simulink library "Cassie_CommandBlock_Library_1"  (R2017b)
settings: Solver=VariableStepAuto  StartTime=0.0  StopTime=10.0  RelTol=1e-3
undefined symbols (not defined in the file): isSim, UserParams
settings Model: Creator=81068  LastModifiedBy=81068

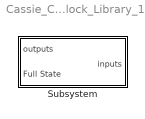
== system Cassie_CommandBlock_Library_1 ==
  Subsystem : Subsystem

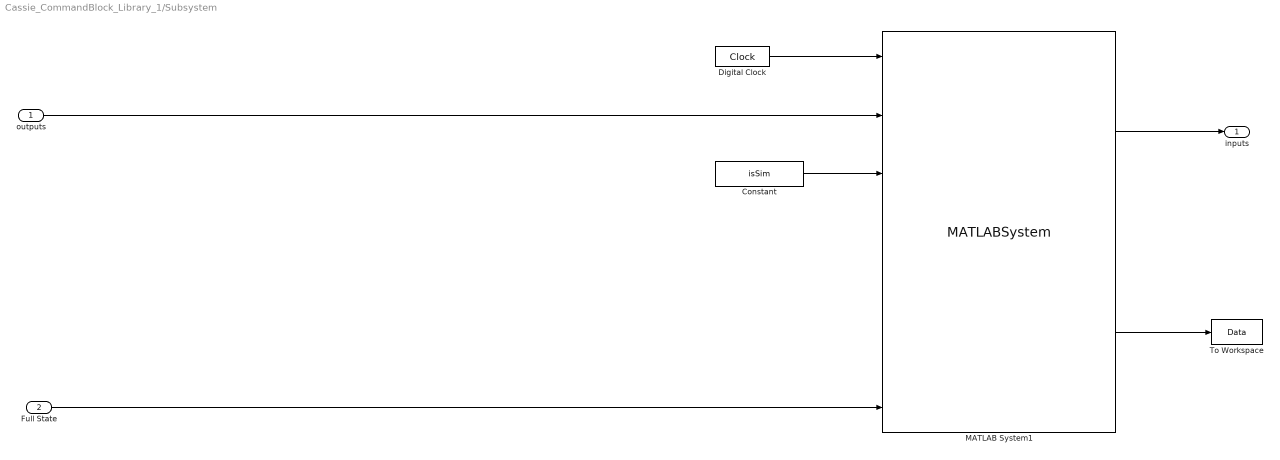
== system Cassie_CommandBlock_Library_1/Subsystem ==
  outputs : Inport  OutDataTypeStr=Bus: CassieOutBus
  Full State : Inport  Port=2
  Constant : Constant  Value=isSim  OutDataTypeStr=int8  LockScale=on
  Digital Clock : DigitalClock  SampleTime=UserParams.SampleTime
  MATLAB System1 : MATLABSystem  System=Cassie_Controller_1  SimulateUsing=Code generation
      mask Type: Cassie_Controller_1
      mask Display:
      | disp('Cassie_Controller_1');
      | port_label('output',1,'userInputs');
      | port_label('output',2,'Data');
  To Workspace : ToWorkspace  VariableName=Data  SaveFormat=Timeseries  SampleTime=-1
  "inputs " : Outport
  wires:
  outputs/1 -> MATLAB System1/2
  MATLAB System1/1 -> "inputs "/1
  MATLAB System1/2 -> To Workspace/1
  Digital Clock/1 -> MATLAB System1/1
  Constant/1 -> MATLAB System1/3
  Full State/1 -> MATLAB System1/7
